simulink model "pcssp_KMAG_wrapper"  (R2021b)
settings: configuration reference "configurationSettings" (kept outside this file)
settings Model: DataDictionary=pcssp_KMAG_wrapper.sldd  Creator=ravenst1  LastModifiedBy=ravenst1
settings ConfigSetRef: SourceName=configurationSettings

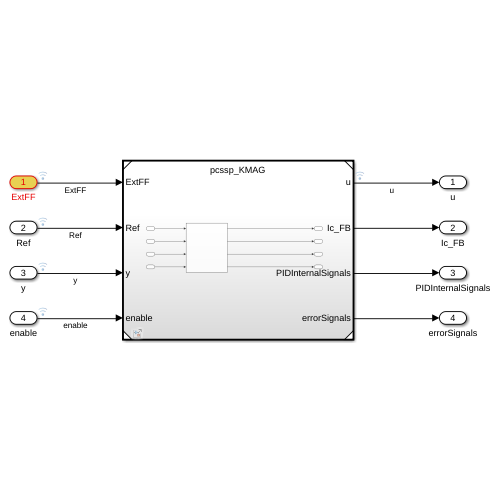
[thumbnail: Simulink's stored preview of the top-level diagram]
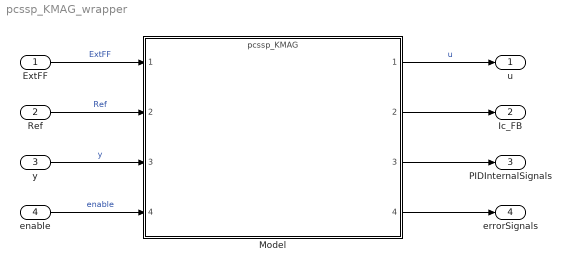
== system pcssp_KMAG_wrapper ==
  ExtFF : Inport  PortDimensions=size_KMAG.extFF
  Ref : Inport  Port=2  PortDimensions=size_KMAG.Ref
  y : Inport  Port=3  PortDimensions=size_KMAG.y
  enable : Inport  Port=4  PortDimensions=size_KMAG.enable
  Model : ModelReference  ModelNameDialog=pcssp_KMAG.slx  SimulationMode=Normal  ModelReferenceVersion=3.2
  u : Outport
  Ic_FB : Outport  Port=2
  PIDInternalSignals : Outport  Port=3
  errorSignals : Outport  Port=4
  wires:
  ExtFF/1 -> Model/1  "ExtFF"
  enable/1 -> Model/4  "enable"
  y/1 -> Model/3  "y"
  Ref/1 -> Model/2  "Ref"
  Model/1 -> u/1  "u"
  Model/2 -> Ic_FB/1
  Model/3 -> PIDInternalSignals/1
  Model/4 -> errorSignals/1
